simulink model "parallel"  (R2021b)
settings: Solver=VariableStepAuto  StartTime=0.0  StopTime=15  RelTol=1e-3
undefined symbols (not defined in the file): fd, invMd, K, KD, KF, KI, KP, Md, xd, xr
settings Model: Creator=simon  LastModifiedBy=buse
settings SolverCC: AlgebraicLoopSolver=TrustRegion
settings DebuggingCC: SFMachineParentedDataDiag=warning

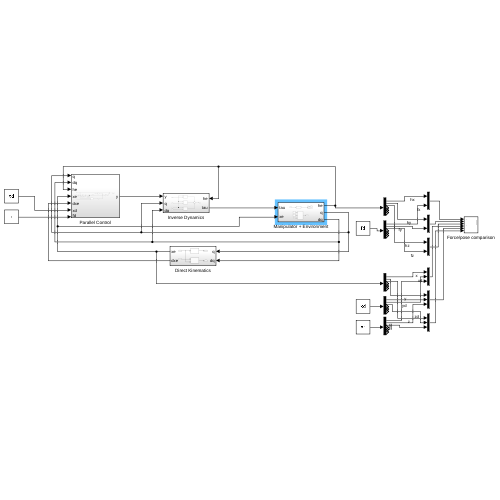
[thumbnail: Simulink's stored preview of the top-level diagram]
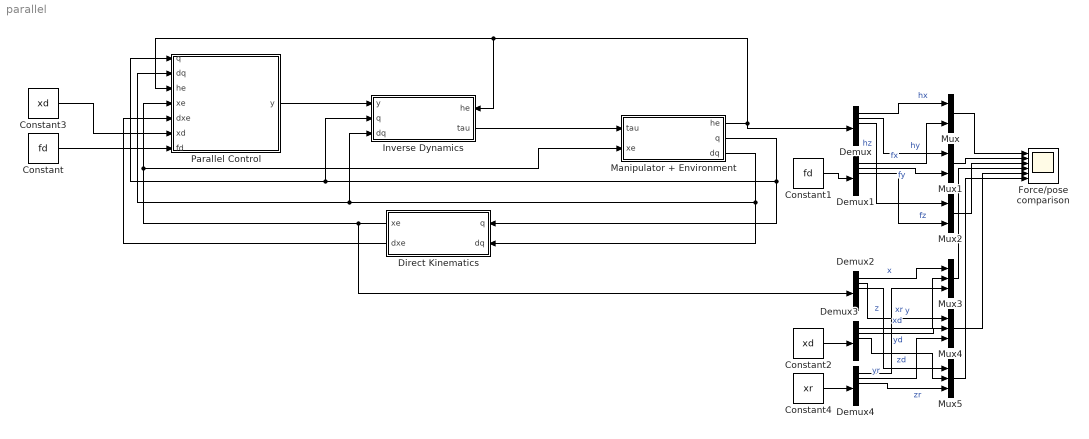
== system parallel ==
  Constant : Constant  Value=fd
  Constant1 : Constant  Value=fd
  Constant2 : Constant  Value=xd
  Constant3 : Constant  Value=xd
  Constant4 : Constant  Value=xr
  Demux{,1..4} (5 alike) : Demux  Outputs=6
  Direct Kinematics : Subsystem
  Force/pose comparison : Scope  NumInputPorts=6
  Inverse Dynamics : Subsystem
      settings: PortSchema="{\"entries\":[{\"content\":{\"sides\":[{\"content\":{\"connectorIds\":[\"In1\",\"In2\",\"In3\"]},\"type\":\"ConnectorPlacement.EquallySpacedRectSide\",\"uuid\":\"ca444f18-8ac7-40fd-b184-99b7b20e73ae\"},{\"content\":{\"connectorIds\":[\"In4\",\"Out1\"],\"side\":\"RIGHT\"},\"type\":\"ConnectorPlacement.EquallySpacedRectSide\",\"uuid\":\"175bb62b-c698-426a-a7ed-7f17edc65a29\"},{\"content\":{\"connectorIds\":[],\"side\":\"TOP\"},\"type\":\"ConnectorPlacement.EquallySpacedRectSide\",\"uuid\":\"77bd2f3a-5c58-46dc-8f82-aed93a477f7f\"}]},\"type\":\"ConnectorPlacement.EquallySpacedConnector\",\"uuid\":\"99286165-21e8-4db9-b2d5-c5081e8b499e\"}],\"packageUris\":[\"http://schema.mathworks.com/mf0/Connector/R2020b\"],\"version\":\"1.0\"}"
  Manipulator + Environment : Subsystem
  Mux : Mux  Inputs=2
  Mux1 : Mux  Inputs=2
  Mux2 : Mux  Inputs=2
  Mux3 : Mux  Inputs=3
  Mux4 : Mux  Inputs=3
  Mux5 : Mux  Inputs=3
  Parallel Control : Subsystem
  wires:
  Inverse Dynamics/1(tau) -> Manipulator + Environment/1(tau)
  Manipulator + Environment/2(q) -> Parallel Control/1(q), Inverse Dynamics/2(q), Direct Kinematics/1(q)
  Manipulator + Environment/3(dq) -> Direct Kinematics/2(dq), Parallel Control/2(dq), Inverse Dynamics/3(dq)
  Direct Kinematics/1(xe) -> Demux2/1, Parallel Control/4(xe), Manipulator + Environment/2(xe)
  Parallel Control/1(y) -> Inverse Dynamics/1(y)
  Direct Kinematics/2(dxe) -> Parallel Control/5(dxe)
  Constant/1 -> Parallel Control/7(fd)
  Manipulator + Environment/1(he) -> Demux/1, Parallel Control/3(he), Inverse Dynamics/4(he)
  Constant1/1 -> Demux1/1
  Demux/1 -> Mux/1  "hx"
  Demux/2 -> Mux1/1  "hy"
  Demux/3 -> Mux2/1  "hz"
  Demux1/1 -> Mux/2  "fx"
  Demux1/2 -> Mux1/2  "fy"
  Demux1/3 -> Mux2/2  "fz"
  Mux/1 -> Force/pose comparison/1
  Mux1/1 -> Force/pose comparison/2
  Mux2/1 -> Force/pose comparison/3
  Demux2/1 -> Mux3/1  "x"
  Mux4/1 -> Force/pose comparison/5
  Mux3/1 -> Force/pose comparison/4
  Demux3/1 -> Mux3/2  "xd"
  Demux2/3 -> Mux5/1  "z"
  Mux5/1 -> Force/pose comparison/6
  Demux3/2 -> Mux4/2  "yd"
  Demux3/3 -> Mux5/2  "zd"
  Demux2/2 -> Mux4/1  "y"
  Constant2/1 -> Demux3/1
  Constant3/1 -> Parallel Control/6(xd)
  Constant4/1 -> Demux4/1
  Demux4/1 -> Mux3/3  "xr"
  Demux4/2 -> Mux4/3  "yr"
  Demux4/3 -> Mux5/3  "zr"

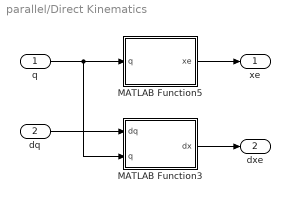
== system parallel/Direct Kinematics ==
  q : Inport
  dq : Inport  Port=2
  MATLAB Function3 : MATLAB Function  TreatAsAtomicUnit=on
  MATLAB Function5 : MATLAB Function  TreatAsAtomicUnit=on
  xe : Outport
  dxe : Outport  Port=2
  wires:
  MATLAB Function3/1(dx) -> dxe/1
  q/1 -> MATLAB Function3/2(q), MATLAB Function5/1(q)
  MATLAB Function5/1(xe) -> xe/1
  dq/1 -> MATLAB Function3/1(dq)

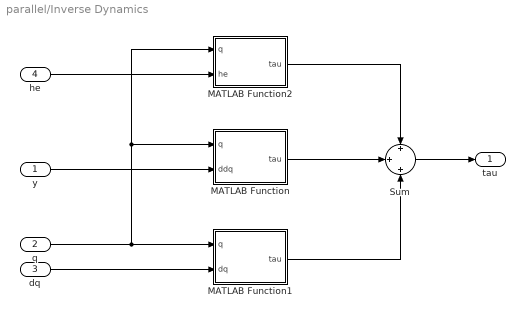
== system parallel/Inverse Dynamics ==
  y : Inport
  q : Inport  Port=2
  dq : Inport  Port=3
  he : Inport  Port=4
  MATLAB Function : MATLAB Function  TreatAsAtomicUnit=on
  MATLAB Function1 : MATLAB Function  TreatAsAtomicUnit=on
  MATLAB Function2 : MATLAB Function  TreatAsAtomicUnit=on
  Sum : Sum  Inputs=+|+|+
  tau : Outport
  wires:
  Sum/1 -> tau/1
  dq/1 -> MATLAB Function1/2(dq)
  q/1 -> MATLAB Function/1(q), MATLAB Function2/1(q), MATLAB Function1/1(q)
  y/1 -> MATLAB Function/2(ddq)
  he/1 -> MATLAB Function2/2(he)
  MATLAB Function2/1(tau) -> Sum/1
  MATLAB Function/1(tau) -> Sum/2
  MATLAB Function1/1(tau) -> Sum/3

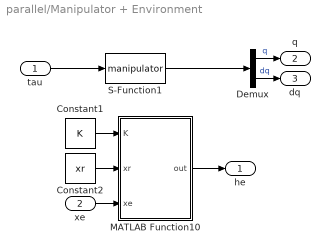
== system parallel/Manipulator + Environment ==
  tau : Inport
  xe : Inport  Port=2
  Constant1 : Constant  Value=K
  Constant2 : Constant  Value=xr
  Demux : Demux  Outputs=2
  MATLAB Function10 : MATLAB Function  TreatAsAtomicUnit=on
  S-Function1 : S-Function  FunctionName=manipulator  Parameters=robot  SFunctionDeploymentMode=off  EnableBusSupport=off
  he : Outport
  q : Outport  Port=2
  dq : Outport  Port=3
  wires:
  tau/1 -> S-Function1/1
  Constant1/1 -> MATLAB Function10/1(K)
  Constant2/1 -> MATLAB Function10/2(xr)
  xe/1 -> MATLAB Function10/3(xe)
  S-Function1/1 -> Demux/1
  Demux/1 -> q/1  "q"
  Demux/2 -> dq/1  "dq"
  MATLAB Function10/1(out) -> he/1

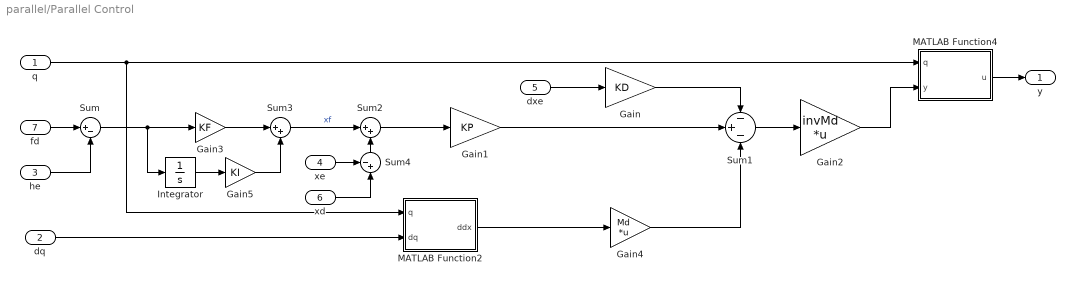
== system parallel/Parallel Control ==
  q : Inport
  dq : Inport  Port=2
  he : Inport  Port=3
  xe : Inport  Port=4
  dxe : Inport  Port=5
  xd : Inport  Port=6
  fd : Inport  Port=7
  Gain : Gain  Gain=KD
  Gain1 : Gain  Gain=KP
  Gain2 : Gain  Gain=invMd  Multiplication=Matrix(K*u)
  Gain3 : Gain  Gain=KF
  Gain4 : Gain  Gain=Md  Multiplication=Matrix(K*u)
  Gain5 : Gain  Gain=KI
  Integrator : Integrator
  MATLAB Function2 : MATLAB Function  TreatAsAtomicUnit=on
  MATLAB Function4 : MATLAB Function  TreatAsAtomicUnit=on
  Sum : Sum  Inputs=|+-
  Sum1 : Sum  Inputs=-+-
  Sum2 : Sum  Inputs=|++
  Sum3 : Sum  Inputs=|++
  Sum4 : Sum  Inputs=-+|
  y : Outport
  wires:
  Integrator/1 -> Gain5/1
  fd/1 -> Sum/1
  Sum/1 -> Integrator/1, Gain3/1
  dxe/1 -> Gain/1
  Gain/1 -> Sum1/1
  Gain1/1 -> Sum1/2
  MATLAB Function2/1(ddx) -> Gain4/1
  Sum3/1 -> Sum2/1  "xf"
  Gain4/1 -> Sum1/3
  MATLAB Function4/1(u) -> y/1
  q/1 -> MATLAB Function4/1(q), MATLAB Function2/1(q)
  Gain2/1 -> MATLAB Function4/2(y)
  he/1 -> Sum/2
  Gain3/1 -> Sum3/1
  dq/1 -> MATLAB Function2/2(dq)
  Sum2/1 -> Gain1/1
  Gain5/1 -> Sum3/2
  Sum1/1 -> Gain2/1
  Sum4/1 -> Sum2/2
  xe/1 -> Sum4/1
  xd/1 -> Sum4/2

== matlab function parallel/Inverse Dynamics/MATLAB Function1 ==
  data: q input size=3; tau output; dq input size=3
function tau = N(q, dq)
    q1 = q(1); q2 = q(2); q3 = q(3);
    dq1 = dq(1); dq2 = dq(2); dq3 = dq(3);
    tau = [dq3*(0.03923*cos(q3)*dq3^2 - 0.5*dq1*(0.0474*sin(2.0*q3) + 0.05885*sin(q3) + 0.1962*q2*sin(q3))*dq3) - 1.0*dq1*(0.5*dq3^2*(0.0474*sin(2.0*q3) + 0.05885*sin(q3) + 0.1962*q2*sin(q3)) - 0.5*dq2^2*(3.098*q2 + 0.1962*cos(q3) + 0.7099)) + 0.5*dq1*dq2^2*(3.098*q2 + 0.1962*cos(q3) + 0.7099);
            0.5*dq1^2*dq2*(3.098*q2 + 0.1962*cos(q3) + 0.7099);
            dq1*(0.03923*cos(q3)*dq3^2 - 0.5*dq1*(0.0474*sin(2.0*q3) + 0.05885*sin(q3) + 0.1962*q2*sin(q3))*dq3) - 0.9621*cos(q3)];
end

== matlab function parallel/Inverse Dynamics/MATLAB Function ==
  data: q input size=3; tau output; ddq input size=3
function tau = B(q, ddq)
    q1 = q(1); q2 = q(2); q3 = q(3);
    B = getB(q,0);
    tau = B*ddq;

== matlab function parallel/Inverse Dynamics/MATLAB Function2 ==
  data: q input; tau output; he input
function tau = Jt(q,he)
    q1 = q(1); q2 = q(2); q3 = q(3);
    JGt = [[(3*cos(q1))/10 - (2*sin(q1))/5 + (6*cos(q1)*cos(q3))/25 + q2*cos(q1), (2*cos(q1))/5 + (3*sin(q1))/10 + (6*cos(q3)*sin(q1))/25 + q2*sin(q1),              0,        0,        0, 1]
        [                                                             sin(q1),                                                             -cos(q1),              0,        0,        0, 0]
        [                                             -(6*sin(q1)*sin(q3))/25,                                               (6*cos(q1)*sin(q3))/25, (6*cos(q3))/25, -cos(q1), -sin(q1), 0]
         ];
    tau = JGt*he;

== matlab function parallel/Direct Kinematics/MATLAB Function3 ==
  data: dq input; dx output; q input
function dx = JA(dq, q)
    q1 = q(1); q2 = q(2); q3 = q(3);
    JA =[(3*cos(q1))/10 - (2*sin(q1))/5 + (6*cos(q1)*cos(q3))/25 + q2*cos(q1),  sin(q1), -(6*sin(q1)*sin(q3))/25;
        (2*cos(q1))/5 + (3*sin(q1))/10 + (6*cos(q3)*sin(q1))/25 + q2*sin(q1), -cos(q1),  (6*cos(q1)*sin(q3))/25;
        0,        0,          (6*cos(q3))/25;
        1,        0,                       0;
        0,        0,                      -1;
        0,        0,                       0]; 
    dx = JA*dq;

== matlab function parallel/Parallel Control/MATLAB Function2 ==
  data: q input; dq input; ddx output
function ddx = dJA(q,dq)
    q1 = q(1); q2 = q(2); q3 = q(3);
    dq1 = dq(1); dq2 = dq(2); dq3 = dq(3);
    dJA =[dq2*cos(q1) - (2*dq1*cos(q1))/5 - (3*dq1*sin(q1))/10 - dq1*sin(q1)*q2 - (6*dq1*cos(q3)*sin(q1))/25 - (6*dq3*cos(q1)*sin(q3))/25, dq1*cos(q1), - (6*dq1*cos(q1)*sin(q3))/25 - (6*dq3*cos(q3)*sin(q1))/25;
(3*dq1*cos(q1))/10 - (2*dq1*sin(q1))/5 + dq2*sin(q1) + (6*dq1*cos(q1)*cos(q3))/25 - (6*dq3*sin(q1)*sin(q3))/25 + dq1*cos(q1)*q2, dq1*sin(q1),   (6*dq3*cos(q1)*cos(q3))/25 - (6*dq1*sin(q1)*sin(q3))/25;
             0,              0,                                                -(6*dq3*sin(q3))/25;
             0,              0,                                                                     0;
             0,              0,                                                                     0;
             0,              0,                                                                     0];
    ddx = dJA*dq;

== matlab function parallel/Direct Kinematics/MATLAB Function5 ==
  data: q input size=3; xe output size=6
function xe = k(q)
    q1 = q(1); q2 = q(2); q3 = q(3);
    % Direct kinematics
    xe = [(2*cos(q1))/5 + (3*sin(q1))/10 + (6*cos(q3)*sin(q1))/25 + q2*sin(q1);
         (2*sin(q1))/5 - (3*cos(q1))/10 - (6*cos(q1)*cos(q3))/25 - q2*cos(q1);
         (6*sin(q3))/25 + 3/20;
         q1;
         pi/2 - q3;
         pi/2];

== matlab function parallel/Parallel Control/MATLAB Function4 ==
  data: q input; y input; u output
function u = invJA(q,y)
    q1 = q(1); q2 = q(2); q3 = q(3);
    JAinv =  [
[                                                                                                                                                             (10.0*cos(q1)*(1.0e+33*q2 + 2.4e+32*cos(q3) + 3.0e+32))/(6.0e+33*q2 + 1.44e+33*cos(q3) + 5.76e+32*cos(q3)^2 + 4.8e+33*q2*cos(q3) + 1.0e+34*q2^2 + 1.09e+34),                                                                                                                                                                         (10.0*sin(q1)*(1.0e+33*q2 + 2.4e+32*cos(q3) + 3.0e+32))/(6.0e+33*q2 + 1.44e+33*cos(q3) + 5.76e+32*cos(q3)^2 + 4.8e+33*q2*cos(q3) + 1.0e+34*q2^2 + 1.09e+34),                                                         0, 1.0e+34/(6.0e+33*q2 + 1.44e+33*cos(q3) + 5.76e+32*cos(q3)^2 + 4.8e+33*q2*cos(q3) + 1.0e+34*q2^2 + 1.09e+34),                                                  0, 0]
[(1.2e+33*cos(q1) + 1.09e+34*sin(q1) + 9.6e+32*cos(q1)*cos(q3) + 1.0e+34*q2^2*sin(q1) + 1.44e+33*cos(q3)*sin(q1) + 5.76e+32*cos(q3)^2*sin(q1) + 4.0e+33*q2*cos(q1) + 6.0e+33*q2*sin(q1) + 4.8e+33*q2*cos(q3)*sin(q1))/(6.0e+33*q2 + 1.44e+33*cos(q3) + 5.76e+32*cos(q3)^2 + 4.8e+33*q2*cos(q3) + 1.0e+34*q2^2 + 1.09e+34), -(1.0e-32*(1.09e+66*cos(q1) - 1.2e+65*sin(q1) + 1.0e+66*q2^2*cos(q1) + 1.44e+65*cos(q1)*cos(q3) - 9.6e+64*cos(q3)*sin(q1) + 5.76e+64*cos(q1)*cos(q3)^2 + 6.0e+65*q2*cos(q1) - 4.0e+65*q2*sin(q1) + 4.8e+65*q2*cos(q1)*cos(q3)))/(6.0e+33*q2 + 1.44e+33*cos(q3) + 5.76e+32*cos(q3)^2 + 4.8e+33*q2*cos(q3) + 1.0e+34*q2^2 + 1.09e+34), (2.88e+32*sin(2.0*q3))/(2.88e+32*cos(2.0*q3) + 1.029e+34), 4.0e+33/(6.0e+33*q2 + 1.44e+33*cos(q3) + 5.76e+32*cos(q3)^2 + 4.8e+33*q2*cos(q3) + 1.0e+34*q2^2 + 1.09e+34), (2.4e+33*sin(q3))/(5.76e+32*sin(q3)^2 - 1.058e+34), 0]
[                                                                                                                                                                                                                                                                                                                       0,                                                                                                                                                                                                                                                                                                                                   0,          (2.4e+33*cos(q3))/(5.76e+32*cos(q3)^2 + 1.0e+34),                                                                                                           0,           1.0e+34/(5.76e+32*sin(q3)^2 - 1.058e+34), 0]];
    u = JAinv*y;

== matlab function parallel/Manipulator + Environment/MATLAB Function10 ==
  data: K input; out output size=6; xr input; xe input size=6
function out = he(K, xr, xe)
    he = zeros(6,1);
    if xe(1) > xr(1) % Only along x, i.e. only when moving only joint 2
        % In contact
        he = K*(xe-xr);
    end
    % Equilibrium point
    out = he;
